simulink model "Ensamble_robot_1"  (R2019b)
settings: Solver=VariableStepAuto  StartTime=0.0  StopTime=10.0  RelTol=1e-3
undefined symbols (not defined in the file or in its folder): Brazo_1, Brazo_2, Ensamble_robot, Pinza, Pinza_1, RootGround, RootPart, Soporte, Torre
libraries: mblibv1 x19
settings Model: Creator=juan  LastModifiedBy=juan
settings SimMechanicsCC: VisOnUpdateDiagram=on  VisDuringSimulation=on

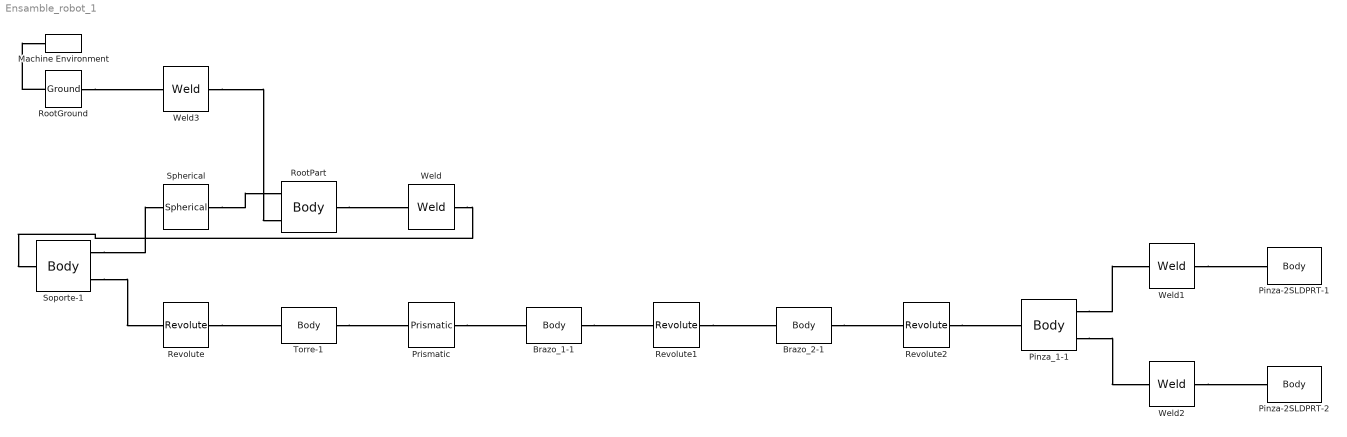
== system Ensamble_robot_1 ==
  Brazo_1-1 : mblibv1/Bodies/Body  LConnTagsString=CS2  RConnTagsString=CS3  UpdateFromCAD=on  PMImportedID=Brazo_1-1  DialogClass=MechanicalBodyBlock  Mass=5.04274  MassUnits=kg  InertiaUnits=kg*m^2  Inertia=[0.0173518,0.0122763,1.33704e-09;0.0122763,0.106444,-1.19326e-09;1.33704e-09,-1.19326e-09,0.102671]  Shape=Cylinder  ShapeDims=[1 1]  ShapeUnits=m  ShapeUse=false  Density=1  DensityUnits=kg/m^3  DensityUse=false  GraphicsMode=GFXFILE  GraphicsFileName=Ensamble_robot - Brazo_1-1.STL  BodyColorSelMode=COLORPALETTE  BodyColor=[1;1;1]  AttachedToCS=CS1  CG=Right$CG$[0.204832 0.0464629 2.69197e-09]$WORLD$WORLD$m$[1 0 0;0 1 0;0 0 1]$3x3 Transform$rad$WORLD$false$Brazo_1-1::CG(AUTOGEN)  WorkingFrames=Right$CS1$[0.45 0.0499751 0]$WORLD$WORLD$m$[1 0 0;0 1 0;0 0 1]$3x3 Transform$rad$WORLD$false$Brazo_1-1::CS1(AUTOGEN)#Left$CS2$[0 0.149975 0.045]$WORLD$WORLD$m$[1 0 0;0 1 0;0 0 1]$3x3 Transform$rad$WORLD$true$Brazo_1-1:-:Torre-1::Brazo_1-1(AUTOGEN)#Right$CS3$[0.45 0.0299751 0]$WORLD$WORLD$m$[1 0 0;0 1 0;0 0 1]$3x3 Transform$rad$WORLD$true$Brazo_1-1:-:Brazo_2-1::Brazo_1-1(AUTOGEN)  CGPos=[0.204832 0.0464629 2.69197e-09]  CGRot=[1 0 0;0 1 0;0 0 1]  CS0Pos=[]  CS0Rot=[]  CS1Pos=[0.45 0.0499751 0]  CS1Rot=[1 0 0;0 1 0;0 0 1]  CS2Pos=[0 0.149975 0.045]  CS2Rot=[1 0 0;0 1 0;0 0 1]  CS3Pos=[0.45 0.0299751 0]  CS3Rot=[1 0 0;0 1 0;0 0 1]  CS4Pos=[]  CS4Rot=[]  CS5Pos=[]  CS5Rot=[]  CS6Pos=[]  CS6Rot=[]  CS7Pos=[]  CS7Rot=[]  CS8Pos=[]  CS8Rot=[]  CS9Pos=[]  CS9Rot=[]  CS10Pos=[]  CS10Rot=[]  CS11Pos=[]  CS11Rot=[]  CS12Pos=[]  CS12Rot=[]  CS13Pos=[]  CS13Rot=[]  CS14Pos=[]  CS14Rot=[]  CS15Pos=[]  CS15Rot=[]  CS16Pos=[]  CS16Rot=[]  CS17Pos=[]  CS17Rot=[]  CS18Pos=[]  CS18Rot=[]  CS19Pos=[]  CS19Rot=[]  CS20Pos=[]  CS20Rot=[]
      settings: SourceProductName=Simscape Multibody  SourceProductBaseCode=MS
  Brazo_2-1 : mblibv1/Bodies/Body  LConnTagsString=CS2  RConnTagsString=CS3  UpdateFromCAD=on  PMImportedID=Brazo_2-1  DialogClass=MechanicalBodyBlock  Mass=1.88667  MassUnits=kg  InertiaUnits=kg*m^2  Inertia=[0.00269492,0.000426403,-1.18231e-09;0.000426403,0.0126019,2.20098e-09;-1.18231e-09,2.20098e-09,0.0117797]  Shape=Cylinder  ShapeDims=[1 1]  ShapeUnits=m  ShapeUse=false  Density=1  DensityUnits=kg/m^3  DensityUse=false  GraphicsMode=GFXFILE  GraphicsFileName=Ensamble_robot - Brazo_2-1.STL  BodyColorSelMode=COLORPALETTE  BodyColor=[1;1;1]  AttachedToCS=CS1  CG=Right$CG$[0.507024 -0.0192513 -1.13579e-08]$WORLD$WORLD$m$[1 0 0;0 1 0;0 0 1]$3x3 Transform$rad$WORLD$false$Brazo_2-1::CG(AUTOGEN)  WorkingFrames=Right$CS1$[0.45 -0.0500249 0]$WORLD$WORLD$m$[1 0 0;0 1 0;0 0 1]$3x3 Transform$rad$WORLD$false$Brazo_2-1::CS1(AUTOGEN)#Left$CS2$[0.45 0.0299751 0]$WORLD$WORLD$m$[1 0 0;0 1 0;0 0 1]$3x3 Transform$rad$WORLD$true$Brazo_1-1:-:Brazo_2-1::Brazo_2-1(AUTOGEN)#Right$CS3$[0.65 -0.0200249 0]$WORLD$WORLD$m$[1 0 0;0 1 0;0 0 1]$3x3 Transform$rad$WORLD$true$Brazo_2-1:-:Pinza_1-1::Brazo_2-1(AUTOGEN)  CGPos=[0.507024 -0.0192513 -1.13579e-08]  CGRot=[1 0 0;0 1 0;0 0 1]  CS0Pos=[]  CS0Rot=[]  CS1Pos=[0.45 -0.0500249 0]  CS1Rot=[1 0 0;0 1 0;0 0 1]  CS2Pos=[0.45 0.0299751 0]  CS2Rot=[1 0 0;0 1 0;0 0 1]  CS3Pos=[0.65 -0.0200249 0]  CS3Rot=[1 0 0;0 1 0;0 0 1]  CS4Pos=[]  CS4Rot=[]  CS5Pos=[]  CS5Rot=[]  CS6Pos=[]  CS6Rot=[]  CS7Pos=[]  CS7Rot=[]  CS8Pos=[]  CS8Rot=[]  CS9Pos=[]  CS9Rot=[]  CS10Pos=[]  CS10Rot=[]  CS11Pos=[]  CS11Rot=[]  CS12Pos=[]  CS12Rot=[]  CS13Pos=[]  CS13Rot=[]  CS14Pos=[]  CS14Rot=[]  CS15Pos=[]  CS15Rot=[]  CS16Pos=[]  CS16Rot=[]  CS17Pos=[]  CS17Rot=[]  CS18Pos=[]  CS18Rot=[]  CS19Pos=[]  CS19Rot=[]  CS20Pos=[]  CS20Rot=[]
      settings: SourceProductName=Simscape Multibody  SourceProductBaseCode=MS
  Machine Environment : mblibv1/Bodies/Machine Environment  PortType=env  PhysicalDomain=Mechanical  DialogTemplateClass=MECH.MachineEnvironment  SyncWhenCopied=off  Gravity=[0 -9.81 0]  GravityUnits=m/s^2  GravityAsSignal=off  Dimensionality=Auto-detect  AnalysisType=Forward dynamics  LinearAssemblyTolerance=1e-3  LinearAssemblyToleranceUnits=m  AngularAssemblyTolerance=1e-3  AngularAssemblyToleranceUnits=rad  ConstraintSolverType=Stabilizing  ConstraintRelTolerance=1e-4  ConstraintAbsTolerance=1e-4  UseRobustSingularityHandling=off  RedundancyAnalysisToleranceType=Automatically select tolerance  RedundancyAnalysisTolerance=1e-14  StatePerturbationType=Fixed  PerturbationSize=1e-5  VisualizeMachine=on  BodyVisualizationType=Use model default body geometries  BodyColorSelMode=Use model default  DefaultBodyColor=[1 0 0]
      settings: SourceProductName=Simscape Multibody  SourceProductBaseCode=MS
  Pinza-2SLDPRT-1 : mblibv1/Bodies/Body  LConnTagsString=CS2  UpdateFromCAD=on  PMImportedID=Pinza-2SLDPRT-1  DialogClass=MechanicalBodyBlock  Mass=0.01755  MassUnits=kg  InertiaUnits=kg*m^2  Inertia=[5.56763e-07,0,0;0,7.2684e-06,0;0,0,6.78476e-06]  Shape=Cylinder  ShapeDims=[1 1]  ShapeUnits=m  ShapeUse=false  Density=1  DensityUnits=kg/m^3  DensityUse=false  GraphicsMode=GFXFILE  GraphicsFileName=Ensamble_robot - Pinza-2SLDPRT-1.STL  BodyColorSelMode=COLORPALETTE  BodyColor=[0.894118;0.913725;0.929412]  AttachedToCS=CS1  CG=Right$CG$[0.705013 -0.0950249 -0.0525]$WORLD$WORLD$m$[1 0 0;0 0 1;0 -1 0]$3x3 Transform$rad$WORLD$false$Pinza-2SLDPRT-1::CG(AUTOGEN)  WorkingFrames=Right$CS1$[0.697 -0.0950249 -0.05]$WORLD$WORLD$m$[1 0 0;0 0 1;0 -1 0]$3x3 Transform$rad$WORLD$false$Pinza-2SLDPRT-1::CS1(AUTOGEN)#Left$CS2$[0.672 -0.105025 -0.055]$WORLD$WORLD$m$[1 0 0;0 1 0;0 0 1]$3x3 Transform$rad$WORLD$true$Pinza-2SLDPRT-1:-:Pinza_1-1::Pinza-2SLDPRT-1(AUTOGEN)  CGPos=[0.705013 -0.0950249 -0.0525]  CGRot=[1 0 0;0 0 1;0 -1 0]  CS0Pos=[]  CS0Rot=[]  CS1Pos=[0.697 -0.0950249 -0.05]  CS1Rot=[1 0 0;0 0 1;0 -1 0]  CS2Pos=[0.672 -0.105025 -0.055]  CS2Rot=[1 0 0;0 1 0;0 0 1]  CS3Pos=[]  CS3Rot=[]  CS4Pos=[]  CS4Rot=[]  CS5Pos=[]  CS5Rot=[]  CS6Pos=[]  CS6Rot=[]  CS7Pos=[]  CS7Rot=[]  CS8Pos=[]  CS8Rot=[]  CS9Pos=[]  CS9Rot=[]  CS10Pos=[]  CS10Rot=[]  CS11Pos=[]  CS11Rot=[]  CS12Pos=[]  CS12Rot=[]  CS13Pos=[]  CS13Rot=[]  CS14Pos=[]  CS14Rot=[]  CS15Pos=[]  CS15Rot=[]  CS16Pos=[]  CS16Rot=[]  CS17Pos=[]  CS17Rot=[]  CS18Pos=[]  CS18Rot=[]  CS19Pos=[]  CS19Rot=[]  CS20Pos=[]  CS20Rot=[]
      settings: SourceProductName=Simscape Multibody  SourceProductBaseCode=MS
  Pinza-2SLDPRT-2 : mblibv1/Bodies/Body  LConnTagsString=CS2  UpdateFromCAD=on  PMImportedID=Pinza-2SLDPRT-2  DialogClass=MechanicalBodyBlock  Mass=0.01755  MassUnits=kg  InertiaUnits=kg*m^2  Inertia=[5.56763e-07,0,0;0,7.2684e-06,0;0,0,6.78476e-06]  Shape=Cylinder  ShapeDims=[1 1]  ShapeUnits=m  ShapeUse=false  Density=1  DensityUnits=kg/m^3  DensityUse=false  GraphicsMode=GFXFILE  GraphicsFileName=Ensamble_robot - Pinza-2SLDPRT-2.STL  BodyColorSelMode=COLORPALETTE  BodyColor=[0.894118;0.913725;0.929412]  AttachedToCS=CS1  CG=Right$CG$[0.705013 -0.0950249 0.0525]$WORLD$WORLD$m$[1 0 0;0 0 -1;0 1 0]$3x3 Transform$rad$WORLD$false$Pinza-2SLDPRT-2::CG(AUTOGEN)  WorkingFrames=Right$CS1$[0.697 -0.0950249 0.05]$WORLD$WORLD$m$[1 0 0;0 0 -1;0 1 0]$3x3 Transform$rad$WORLD$false$Pinza-2SLDPRT-2::CS1(AUTOGEN)#Left$CS2$[0.672 -0.105025 0.055]$WORLD$WORLD$m$[1 0 0;0 1 0;0 0 1]$3x3 Transform$rad$WORLD$true$Pinza-2SLDPRT-2:-:Pinza_1-1::Pinza-2SLDPRT-2(AUTOGEN)  CGPos=[0.705013 -0.0950249 0.0525]  CGRot=[1 0 0;0 0 -1;0 1 0]  CS0Pos=[]  CS0Rot=[]  CS1Pos=[0.697 -0.0950249 0.05]  CS1Rot=[1 0 0;0 0 -1;0 1 0]  CS2Pos=[0.672 -0.105025 0.055]  CS2Rot=[1 0 0;0 1 0;0 0 1]  CS3Pos=[]  CS3Rot=[]  CS4Pos=[]  CS4Rot=[]  CS5Pos=[]  CS5Rot=[]  CS6Pos=[]  CS6Rot=[]  CS7Pos=[]  CS7Rot=[]  CS8Pos=[]  CS8Rot=[]  CS9Pos=[]  CS9Rot=[]  CS10Pos=[]  CS10Rot=[]  CS11Pos=[]  CS11Rot=[]  CS12Pos=[]  CS12Rot=[]  CS13Pos=[]  CS13Rot=[]  CS14Pos=[]  CS14Rot=[]  CS15Pos=[]  CS15Rot=[]  CS16Pos=[]  CS16Rot=[]  CS17Pos=[]  CS17Rot=[]  CS18Pos=[]  CS18Rot=[]  CS19Pos=[]  CS19Rot=[]  CS20Pos=[]  CS20Rot=[]
      settings: SourceProductName=Simscape Multibody  SourceProductBaseCode=MS
  Pinza_1-1 : mblibv1/Bodies/Body  LConnTagsString=CS2  RConnTagsString=CS3|CS4  UpdateFromCAD=on  PMImportedID=Pinza_1-1  DialogClass=MechanicalBodyBlock  Mass=1.1552  MassUnits=kg  InertiaUnits=kg*m^2  Inertia=[0.00139548,9.82419e-05,0;9.82419e-05,0.00107204,0;0,0,0.00130274]  Shape=Cylinder  ShapeDims=[1 1]  ShapeUnits=m  ShapeUse=false  Density=1  DensityUnits=kg/m^3  DensityUse=false  GraphicsMode=GFXFILE  GraphicsFileName=Ensamble_robot - Pinza_1-1.STL  BodyColorSelMode=COLORPALETTE  BodyColor=[0.894118;0.913725;0.929412]  AttachedToCS=CS1  CG=Right$CG$[0.653502 -0.0707388 0]$WORLD$WORLD$m$[1 0 0;0 1 0;0 0 1]$3x3 Transform$rad$WORLD$false$Pinza_1-1::CG(AUTOGEN)  WorkingFrames=Right$CS1$[0.65 -0.110025 0]$WORLD$WORLD$m$[1 0 0;0 1 0;0 0 1]$3x3 Transform$rad$WORLD$false$Pinza_1-1::CS1(AUTOGEN)#Left$CS2$[0.65 -0.0200249 0]$WORLD$WORLD$m$[1 0 0;0 1 0;0 0 1]$3x3 Transform$rad$WORLD$true$Brazo_2-1:-:Pinza_1-1::Pinza_1-1(AUTOGEN)#Right$CS3$[0.672 -0.105025 -0.055]$WORLD$WORLD$m$[1 0 0;0 1 0;0 0 1]$3x3 Transform$rad$WORLD$true$Pinza-2SLDPRT-1:-:Pinza_1-1::Pinza_1-1(AUTOGEN)#Right$CS4$[0.672 -0.105025 0.055]$WORLD$WORLD$m$[1 0 0;0 1 0;0 0 1]$3x3 Transform$rad$WORLD$true$Pinza-2SLDPRT-2:-:Pinza_1-1::Pinza_1-1(AUTOGEN)  CGPos=[0.653502 -0.0707388 0]  CGRot=[1 0 0;0 1 0;0 0 1]  CS0Pos=[]  CS0Rot=[]  CS1Pos=[0.65 -0.110025 0]  CS1Rot=[1 0 0;0 1 0;0 0 1]  CS2Pos=[0.65 -0.0200249 0]  CS2Rot=[1 0 0;0 1 0;0 0 1]  CS3Pos=[0.672 -0.105025 -0.055]  CS3Rot=[1 0 0;0 1 0;0 0 1]  CS4Pos=[0.672 -0.105025 0.055]  CS4Rot=[1 0 0;0 1 0;0 0 1]  CS5Pos=[]  CS5Rot=[]  CS6Pos=[]  CS6Rot=[]  CS7Pos=[]  CS7Rot=[]  CS8Pos=[]  CS8Rot=[]  CS9Pos=[]  CS9Rot=[]  CS10Pos=[]  CS10Rot=[]  CS11Pos=[]  CS11Rot=[]  CS12Pos=[]  CS12Rot=[]  CS13Pos=[]  CS13Rot=[]  CS14Pos=[]  CS14Rot=[]  CS15Pos=[]  CS15Rot=[]  CS16Pos=[]  CS16Rot=[]  CS17Pos=[]  CS17Rot=[]  CS18Pos=[]  CS18Rot=[]  CS19Pos=[]  CS19Rot=[]  CS20Pos=[]  CS20Rot=[]
      settings: SourceProductName=Simscape Multibody  SourceProductBaseCode=MS
  Prismatic : mblibv1/Joints/Prismatic  LConnTagsString=__newl0  RConnTagsString=__newr0  UpdateFromCAD=on  PMImportedID=Brazo_1-1:-:Torre-1  NumSAPorts=0  CutJoint=off  MarkAsCut=off  Primitives=prismatic  PrimitiveProps=P1$WORLD$[0,-1,0]$prismatic  DialogClass=JointBlock  P1Axis=[0,-1,0]
      settings: SourceProductName=Simscape Multibody  SourceProductBaseCode=MS
  Revolute : mblibv1/Joints/Revolute  LConnTagsString=__newl0  RConnTagsString=__newr0  UpdateFromCAD=on  PMImportedID=Soporte-1:-:Torre-1  NumSAPorts=0  CutJoint=off  MarkAsCut=off  Primitives=prismatic  PrimitiveProps=R1$WORLD$[0,1,0]$revolute  DialogClass=JointBlock  R1Axis=[0,1,0]
      settings: SourceProductName=Simscape Multibody  SourceProductBaseCode=MS
  Revolute1 : mblibv1/Joints/Revolute  LConnTagsString=__newl0  RConnTagsString=__newr0  UpdateFromCAD=on  PMImportedID=Brazo_1-1:-:Brazo_2-1  NumSAPorts=0  CutJoint=off  MarkAsCut=off  Primitives=prismatic  PrimitiveProps=R1$WORLD$[0,-1,0]$revolute  DialogClass=JointBlock  R1Axis=[0,-1,0]
      settings: SourceProductName=Simscape Multibody  SourceProductBaseCode=MS
  Revolute2 : mblibv1/Joints/Revolute  LConnTagsString=__newl0  RConnTagsString=__newr0  UpdateFromCAD=on  PMImportedID=Brazo_2-1:-:Pinza_1-1  NumSAPorts=0  CutJoint=off  MarkAsCut=off  Primitives=prismatic  PrimitiveProps=R1$WORLD$[0,-1,0]$revolute  DialogClass=JointBlock  R1Axis=[0,-1,0]
      settings: SourceProductName=Simscape Multibody  SourceProductBaseCode=MS
  RootGround : mblibv1/Bodies/Ground  UpdateFromCAD=on  PMImportedID=RootGround  LeftPortType=env  RightPortType=workingframe  PhysicalDomain=Mechanical  DialogClass=GroundBlock  CoordPosition=[0.0659419,0.00229338,1.11665e-06]  CoordPositionUnits=m  StateVectorMgrId=1  MachineId=[2 0]  ShowEnvPort=on  ParameterChecksum=[2902885215, 1976529096, 3323352035, 3145786115]  TopologyChecksum=[2972919434, 4102682500, 2049195146, 1476810250]
      settings: SourceProductName=Simscape Multibody  SourceProductBaseCode=MS
  RootPart : mblibv1/Bodies/Body  LConnTagsString=CS3|CS4  RConnTagsString=CS2  UpdateFromCAD=on  PMImportedID=Ensamble_robot/RootPart  DialogClass=MechanicalBodyBlock  Mass=0  MassUnits=kg  InertiaUnits=kg*m^2  Inertia=[0,0,0;0,0,0;0,0,0]  Shape=Cylinder  ShapeDims=[1 1]  ShapeUnits=m  ShapeUse=false  Density=1  DensityUnits=kg/m^3  DensityUse=false  GraphicsMode=MACHINE_DEFAULT  BodyColorSelMode=MACHINE_DEFAULT  BodyColor=[1;0;0]  AttachedToCS=CS1  CG=Right$CG$[0.0659419 0.00229338 1.11665e-06]$WORLD$WORLD$m$[1 0 0;0 1 0;0 0 1]$3x3 Transform$rad$WORLD$false$Ensamble_robot/RootPart::CG(AUTOGEN)  WorkingFrames=Right$CS1$[0 0 0]$WORLD$WORLD$m$[1 0 0;0 1 0;0 0 1]$3x3 Transform$rad$WORLD$false$Ensamble_robot/RootPart::CS1(AUTOGEN)#Right$CS2$[-0.119346 -0.242891 4.53911e-06]$WORLD$WORLD$m$[1 0 0;0 1 0;0 0 1]$3x3 Transform$rad$WORLD$true$Ensamble_robot/RootPart:-:Soporte-1::Ensamble_robot/RootPart(AUTOGEN)#Left$CS3$[0 0 0]$WORLD$WORLD$m$[1 0 0;0 1 0;0 0 1]$3x3 Transform$rad$WORLD$true$:-:Ensamble_robot/RootPart::Ensamble_robot/RootPart(AUTOGEN)#Left$CS4$[0.0659419 0.00229338 1.11665e-06]$WORLD$WORLD$m$[1 0 0;0 1 0;0 0 1]$3x3 Transform$rad$WORLD$true$Ensamble_robot/RootPart:-:RootGround::Ensamble_robot/RootPart(AUTOGEN)  CGPos=[0.0659419 0.00229338 1.11665e-06]  CGRot=[1 0 0;0 1 0;0 0 1]  CS0Pos=[]  CS0Rot=[]  CS1Pos=[0 0 0]  CS1Rot=[1 0 0;0 1 0;0 0 1]  CS2Pos=[-0.119346 -0.242891 4.53911e-06]  CS2Rot=[1 0 0;0 1 0;0 0 1]  CS3Pos=[0 0 0]  CS3Rot=[1 0 0;0 1 0;0 0 1]  CS4Pos=[0.0659419 0.00229338 1.11665e-06]  CS4Rot=[1 0 0;0 1 0;0 0 1]  CS5Pos=[]  CS5Rot=[]  CS6Pos=[]  CS6Rot=[]  CS7Pos=[]  CS7Rot=[]  CS8Pos=[]  CS8Rot=[]  CS9Pos=[]  CS9Rot=[]  CS10Pos=[]  CS10Rot=[]  CS11Pos=[]  CS11Rot=[]  CS12Pos=[]  CS12Rot=[]  CS13Pos=[]  CS13Rot=[]  CS14Pos=[]  CS14Rot=[]  CS15Pos=[]  CS15Rot=[]  CS16Pos=[]  CS16Rot=[]  CS17Pos=[]  CS17Rot=[]  CS18Pos=[]  CS18Rot=[]  CS19Pos=[]  CS19Rot=[]  CS20Pos=[]  CS20Rot=[]
      settings: SourceProductName=Simscape Multibody  SourceProductBaseCode=MS
  Soporte-1 : mblibv1/Bodies/Body  LConnTagsString=CS2  RConnTagsString=CS3|CS4  UpdateFromCAD=on  PMImportedID=Soporte-1  DialogClass=MechanicalBodyBlock  Mass=6.83887  MassUnits=kg  InertiaUnits=kg*m^2  Inertia=[0.0271292,0.00214532,-1.0763e-06;0.00214532,0.102791,-1.48243e-06;-1.0763e-06,-1.48243e-06,0.0878129]  Shape=Cylinder  ShapeDims=[1 1]  ShapeUnits=m  ShapeUse=false  Density=1  DensityUnits=kg/m^3  DensityUse=false  GraphicsMode=GFXFILE  GraphicsFileName=Ensamble_robot - Soporte-1.STL  BodyColorSelMode=COLORPALETTE  BodyColor=[1;1;1]  AttachedToCS=CS1  CG=Right$CG$[-0.119346 -0.242891 4.53911e-06]$WORLD$WORLD$m$[1 0 0;0 1 0;0 0 1]$3x3 Transform$rad$WORLD$false$Soporte-1::CG(AUTOGEN)  WorkingFrames=Right$CS1$[0 -0.29 0]$WORLD$WORLD$m$[1 0 0;0 1 0;0 0 1]$3x3 Transform$rad$WORLD$false$Soporte-1::CS1(AUTOGEN)#Left$CS2$[-0.119346 -0.242891 4.53911e-06]$WORLD$WORLD$m$[1 0 0;0 1 0;0 0 1]$3x3 Transform$rad$WORLD$true$Ensamble_robot/RootPart:-:Soporte-1::Soporte-1(AUTOGEN)#Right$CS3$[0 0 0]$WORLD$WORLD$m$[1 0 0;0 1 0;0 0 1]$3x3 Transform$rad$WORLD$true$:-:Ensamble_robot/RootPart::Soporte-1(AUTOGEN)#Right$CS4$[0 -0.23 0]$WORLD$WORLD$m$[1 0 0;0 1 0;0 0 1]$3x3 Transform$rad$WORLD$true$Soporte-1:-:Torre-1::Soporte-1(AUTOGEN)  CGPos=[-0.119346 -0.242891 4.53911e-06]  CGRot=[1 0 0;0 1 0;0 0 1]  CS0Pos=[]  CS0Rot=[]  CS1Pos=[0 -0.29 0]  CS1Rot=[1 0 0;0 1 0;0 0 1]  CS2Pos=[-0.119346 -0.242891 4.53911e-06]  CS2Rot=[1 0 0;0 1 0;0 0 1]  CS3Pos=[0 0 0]  CS3Rot=[1 0 0;0 1 0;0 0 1]  CS4Pos=[0 -0.23 0]  CS4Rot=[1 0 0;0 1 0;0 0 1]  CS5Pos=[]  CS5Rot=[]  CS6Pos=[]  CS6Rot=[]  CS7Pos=[]  CS7Rot=[]  CS8Pos=[]  CS8Rot=[]  CS9Pos=[]  CS9Rot=[]  CS10Pos=[]  CS10Rot=[]  CS11Pos=[]  CS11Rot=[]  CS12Pos=[]  CS12Rot=[]  CS13Pos=[]  CS13Rot=[]  CS14Pos=[]  CS14Rot=[]  CS15Pos=[]  CS15Rot=[]  CS16Pos=[]  CS16Rot=[]  CS17Pos=[]  CS17Rot=[]  CS18Pos=[]  CS18Rot=[]  CS19Pos=[]  CS19Rot=[]  CS20Pos=[]  CS20Rot=[]
      settings: SourceProductName=Simscape Multibody  SourceProductBaseCode=MS
  Spherical : mblibv1/Joints/Spherical  LConnTagsString=__newl0  RConnTagsString=__newr0  UpdateFromCAD=on  PMImportedID=:-:Ensamble_robot/RootPart  NumSAPorts=0  CutJoint=off  MarkAsCut=off  Primitives=spherical  PrimitiveProps=S$WORLD$[0,0,0]$spherical  DialogClass=JointBlock  SAxis=[0,0,0]
      settings: SourceProductName=Simscape Multibody  SourceProductBaseCode=MS
  Torre-1 : mblibv1/Bodies/Body  LConnTagsString=CS2  RConnTagsString=CS3  UpdateFromCAD=on  PMImportedID=Torre-1  DialogClass=MechanicalBodyBlock  Mass=12.906  MassUnits=kg  InertiaUnits=kg*m^2  Inertia=[0.653453,0.0144429,-5.6767e-09;0.0144429,0.0391342,-1.12795e-08;-5.6767e-09,-1.12795e-08,0.64837]  Shape=Cylinder  ShapeDims=[1 1]  ShapeUnits=m  ShapeUse=false  Density=1  DensityUnits=kg/m^3  DensityUse=false  GraphicsMode=GFXFILE  GraphicsFileName=Ensamble_robot - Torre-1.STL  BodyColorSelMode=COLORPALETTE  BodyColor=[1;1;1]  AttachedToCS=CS1  CG=Right$CG$[-0.00895228 0.124909 6.2308e-09]$WORLD$WORLD$m$[1 0 0;0 1 0;0 0 1]$3x3 Transform$rad$WORLD$false$Torre-1::CG(AUTOGEN)  WorkingFrames=Right$CS1$[0 -0.18 0]$WORLD$WORLD$m$[1 0 0;0 1 0;0 0 1]$3x3 Transform$rad$WORLD$false$Torre-1::CS1(AUTOGEN)#Left$CS2$[0 -0.23 0]$WORLD$WORLD$m$[1 0 0;0 1 0;0 0 1]$3x3 Transform$rad$WORLD$true$Soporte-1:-:Torre-1::Torre-1(AUTOGEN)#Right$CS3$[0 0.5 0.045]$WORLD$WORLD$m$[1 0 0;0 1 0;0 0 1]$3x3 Transform$rad$WORLD$true$Brazo_1-1:-:Torre-1::Torre-1(AUTOGEN)  CGPos=[-0.00895228 0.124909 6.2308e-09]  CGRot=[1 0 0;0 1 0;0 0 1]  CS0Pos=[]  CS0Rot=[]  CS1Pos=[0 -0.18 0]  CS1Rot=[1 0 0;0 1 0;0 0 1]  CS2Pos=[0 -0.23 0]  CS2Rot=[1 0 0;0 1 0;0 0 1]  CS3Pos=[0 0.5 0.045]  CS3Rot=[1 0 0;0 1 0;0 0 1]  CS4Pos=[]  CS4Rot=[]  CS5Pos=[]  CS5Rot=[]  CS6Pos=[]  CS6Rot=[]  CS7Pos=[]  CS7Rot=[]  CS8Pos=[]  CS8Rot=[]  CS9Pos=[]  CS9Rot=[]  CS10Pos=[]  CS10Rot=[]  CS11Pos=[]  CS11Rot=[]  CS12Pos=[]  CS12Rot=[]  CS13Pos=[]  CS13Rot=[]  CS14Pos=[]  CS14Rot=[]  CS15Pos=[]  CS15Rot=[]  CS16Pos=[]  CS16Rot=[]  CS17Pos=[]  CS17Rot=[]  CS18Pos=[]  CS18Rot=[]  CS19Pos=[]  CS19Rot=[]  CS20Pos=[]  CS20Rot=[]
      settings: SourceProductName=Simscape Multibody  SourceProductBaseCode=MS
  Weld : mblibv1/Joints/Weld  LConnTagsString=__newl0  RConnTagsString=__newr0  UpdateFromCAD=on  PMImportedID=Ensamble_robot/RootPart:-:Soporte-1  NumSAPorts=0  CutJoint=off  MarkAsCut=off  Primitives=weld  PrimitiveProps=W$WORLD$[0.57735,0.57735,0.57735]$weld  DialogClass=JointBlock  WAxis=[0.57735,0.57735,0.57735]
      settings: SourceProductName=Simscape Multibody  SourceProductBaseCode=MS
  Weld1 : mblibv1/Joints/Weld  LConnTagsString=__newl0  RConnTagsString=__newr0  UpdateFromCAD=on  PMImportedID=Pinza-2SLDPRT-1:-:Pinza_1-1  NumSAPorts=0  CutJoint=off  MarkAsCut=off  Primitives=weld  PrimitiveProps=W$WORLD$[0.57735,0.57735,0.57735]$weld  DialogClass=JointBlock  WAxis=[0.57735,0.57735,0.57735]
      settings: SourceProductName=Simscape Multibody  SourceProductBaseCode=MS
  Weld2 : mblibv1/Joints/Weld  LConnTagsString=__newl0  RConnTagsString=__newr0  UpdateFromCAD=on  PMImportedID=Pinza-2SLDPRT-2:-:Pinza_1-1  NumSAPorts=0  CutJoint=off  MarkAsCut=off  Primitives=weld  PrimitiveProps=W$WORLD$[0.57735,0.57735,0.57735]$weld  DialogClass=JointBlock  WAxis=[0.57735,0.57735,0.57735]
      settings: SourceProductName=Simscape Multibody  SourceProductBaseCode=MS
  Weld3 : mblibv1/Joints/Weld  LConnTagsString=__newl0  RConnTagsString=__newr0  UpdateFromCAD=on  PMImportedID=Ensamble_robot/RootPart:-:RootGround  NumSAPorts=0  CutJoint=off  MarkAsCut=off  Primitives=weld  PrimitiveProps=W$WORLD$[0.57735,0.57735,0.57735]$weld  DialogClass=JointBlock  WAxis=[0.57735,0.57735,0.57735]
      settings: SourceProductName=Simscape Multibody  SourceProductBaseCode=MS
  connections:
  RootPart/RConn1 -- Weld/LConn1
  Weld/RConn1 -- Soporte-1/LConn1
  Soporte-1/RConn1 -- Spherical/LConn1
  Spherical/RConn1 -- RootPart/LConn1
  Soporte-1/RConn2 -- Revolute/LConn1
  Revolute/RConn1 -- Torre-1/LConn1
  Torre-1/RConn1 -- Prismatic/LConn1
  Prismatic/RConn1 -- Brazo_1-1/LConn1
  Brazo_1-1/RConn1 -- Revolute1/LConn1
  Revolute1/RConn1 -- Brazo_2-1/LConn1
  Brazo_2-1/RConn1 -- Revolute2/LConn1
  Revolute2/RConn1 -- Pinza_1-1/LConn1
  Pinza_1-1/RConn1 -- Weld1/LConn1
  Weld1/RConn1 -- Pinza-2SLDPRT-1/LConn1
  Pinza_1-1/RConn2 -- Weld2/LConn1
  Weld2/RConn1 -- Pinza-2SLDPRT-2/LConn1
  RootGround/RConn1 -- Weld3/LConn1
  Weld3/RConn1 -- RootPart/LConn2
  RootGround/LConn1 -- Machine Environment/RConn1
